simulink model "Traffic_Light_ROS2_demo"  (R2024b)
settings: Solver=FixedStepAuto  StartTime=0.0  StopTime=60  FixedStep=0.1  MaxStep=0.05  RelTol=1e-3
model workspace (MAT data in the model file):
  SL_ROS_VariableLengthArrays_MaxSizes : object (value not decoded)
undefined symbols (not defined in the file or in its folder): brake, gear, hand_brake, manual_gear_shift, reverse, steer, throttle
libraries: ros2lib x9, visionsinks x1
(part 2 of 2)

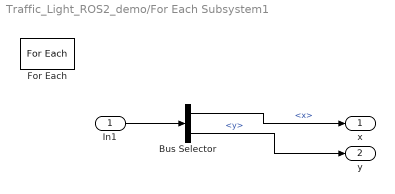
== system Traffic_Light_ROS2_demo/For Each Subsystem1 ==
  In1 : Inport  Partition=on  PartitionDimension=1  PartitionWidth=1  PartitionOffset=0
  Bus Selector : BusSelector  OutputSignals=pose.position.x,pose.position.y
  For Each : ForEach  DisableCoverage=on
  x : Outport  ConcatenationDimension=1
  y : Outport  Port=2  ConcatenationDimension=1
  wires:
  In1/1 -> Bus Selector/1
  Bus Selector/1 -> x/1  "<x>"
  Bus Selector/2 -> y/1  "<y>"

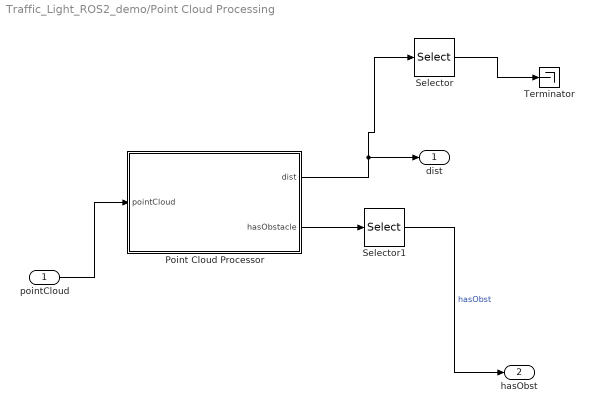
== system Traffic_Light_ROS2_demo/Point Cloud Processing ==
  pointCloud : Inport
  Point Cloud Processor : MATLAB Function  TreatAsAtomicUnit=on
  Selector : Selector  InputPortWidth=10000  IndexOptions=Index vector (dialog)  Indices=1  OutputSizes=1
  Selector1 : Selector  IndexOptions=Index vector (dialog)  Indices=1  OutputSizes=1
  Terminator : Terminator
  dist : Outport
  hasObst : Outport  Port=2
  wires:
  Point Cloud Processor/2(hasObstacle) -> Selector1/1
  Selector/1 -> Terminator/1
  pointCloud/1 -> Point Cloud Processor/1(pointCloud)
  Point Cloud Processor/1(dist) -> dist/1, Selector/1
  Selector1/1 -> hasObst/1  "hasObst"

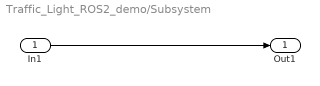
== system Traffic_Light_ROS2_demo/Subsystem ==
  In1 : Inport
  Out1 : Outport
  wires:
  In1/1 -> Out1/1

== matlab function Traffic_Light_ROS2_demo/Point Cloud Processing/Point Cloud Processor ==
  data: pointCloud input; dist output size=[10000,1]; hasObstacle output double
function [dist, hasObstacle] = detectObstacles(pointCloud)
% Detect obstacles from a point cloud and calculate the closest distance.

% Inputs:
%   pointCloud - Nx3 array of [x, y, z] points (point cloud data)
%   lateralRange - Lateral range of interest (meters)
%   zGroundThreshold - Minimum z-value to exclude ground points (meters)

% Outputs:
%   dist - Closest distance to an obstacle (scalar, meters)
%   hasObstacle - Boolean flag indicating if an obstacle is detected

% Initialize outputs
dist = single(inf); % Default to infinity
hasObstacle = 0;


% Check if pointCloud is empty
if isempty(pointCloud)
    return; % Return default outputs
end

% Extract coordinates
x = pointCloud(:, 1); % Forward (X) axis
y = pointCloud(:, 2); % Lateral (Y) axis
z = pointCloud(:, 3); % Vertical (Z) axis

lateralRange = 3;
zGroundThreshold = -2;

% Filter points within region of interest (ROI)
% ROI Criteria:
% - In front of the ego vehicle: x > 0
% - Within lateral range: |y| < lateralRange
% - Above ground: z > zGroundThreshold
isInROI = (x > 0) & (abs(y) < lateralRange) & (z > zGroundThreshold);

% Apply filter
filteredPoints = pointCloud(isInROI, :);

% Compute the closest distance
if ~isempty(filteredPoints)
    % Compute Euclidean distances in the X-Y plane
    % distances = sqrt(filteredPoints(:, 1).^2 + filteredPoints(:, 2).^2); 
    % dist = min(distances); % Find the closest distance
    dist = mean(filteredPoints(:, 1));
    hasObstacle = 1; % Set obstacle flag to true
end

end

== matlab function Traffic_Light_ROS2_demo/Visualize Point cloud2 ==
  data: xyzPoints input
function VisualizePointCloud(xyzPoints)
%VisualizePointCloud Display point cloud

coder.extrinsic('isOpen', 'pcplayer')

persistent player;

if isempty(player)
    % Configure axes limits
    xlimits = [-90 90];
    ylimits = [-90 90];
    zlimits = [ -5 40];
    
    % Create a streaming Lidar viewer
    player = pcplayer(xlimits, ylimits, zlimits);
end

if ~isempty(player) && isOpen(player)
    view(player, xyzPoints);
end

== matlab function Traffic_Light_ROS2_demo/MATLAB Function3 ==
  data: waypointsX input; waypointsX_local output; waypointsY input; vehicleX input; vehicleY input; vehicleYaw input; waypointsY_local output; Curvature output; CurvatureDerivative output; HeadingAngle output; LateralOffset output
function [waypointsX_local, waypointsY_local, Curvature, CurvatureDerivative, HeadingAngle, LateralOffset] = computeLaneCenter(waypointsX, waypointsY, vehicleX, vehicleY, vehicleYaw)
    % Inputs:
    %   waypointsX: X coordinates of the waypoints (Nx1 vector)
    %   waypointsY: Y coordinates of the waypoints (Nx1 vector)
    %   vehicleX: X coordinate of the vehicle
    %   vehicleY: Y coordinate of the vehicle
    %   vehicleYaw: Vehicle orientation (yaw) in radians
    % Outputs:
    %   Curvature: Lane curvature at the vehicle's position
    %   CurvatureDerivative: Rate of change of curvature
    %   HeadingAngle: Lane heading angle at the vehicle's position
    %   LateralOffset: Distance from the vehicle to the lane center (meters)

    % Ensure inputs are column vectors
    waypointsX = waypointsX(:);
    waypointsY = waypointsY(:);

    % Transform waypoints to local vehicle coordinates
    dx = waypointsX - vehicleX;
    dy = waypointsY - vehicleY;
    waypointsX_local = dx * cos(vehicleYaw) + dy * sin(vehicleYaw);
    waypointsY_local = -dx * sin(vehicleYaw) + dy * cos(vehicleYaw);

    % Filter waypoints to include only those ahead of the vehicle
    maxRange = 25; % Limit to 50 meters ahead
    rangeIdx = waypointsX_local > 0 & waypointsX_local < maxRange;
    waypointsX_local = waypointsX_local(rangeIdx);
    waypointsY_local = waypointsY_local(rangeIdx);

    % Ensure enough points are available for fitting
    if numel(waypointsX_local) < 3
        % Not enough points to compute reliably
        Curvature = single(0);
        CurvatureDerivative = single(0);
        HeadingAngle = single(0);
        LateralOffset = single(0);
        return;
    end

    % Fit a 2nd-order polynomial to the filtered waypoints
    polyCoeffs = polyfit(waypointsX_local, waypointsY_local, 2); % y = ax^2 + bx + c
    a = polyCoeffs(1); % Quadratic coefficient
    b = polyCoeffs(2); % Linear coefficient
    c = polyCoeffs(3); % Constant term

    % Curvature: k = 2a / (1 + b^2)^(3/2)
    Curvature = single(2 * a / (1 + b^2)^(3/2));

    % Curvature Derivative: k' = -6a^2b / (1 + b^2)^(5/2)
    CurvatureDerivative = single(-6 * a^2 * b / (1 + b^2)^(5/2));

    % Heading Angle: theta = atan(b)
    HeadingAngle = single(atan(b));

    % Lateral Offset: y = ax^2 + bx + c at x = 0
    LateralOffset = single(c); % Since x_vehicle_local = 0
    % 
    % % Debugging Outputs (optional)
    % disp('Polynomial Coefficients (a, b, c):');
    % disp(polyCoeffs);
    % disp('Curvature:');
    % disp(Curvature);
    % disp('Curvature Derivative:');
    % disp(CurvatureDerivative);
    % disp('Heading Angle:');
    % disp(HeadingAngle);
    % disp('Lateral Offset:');
    % disp(LateralOffset);
end

== matlab function Traffic_Light_ROS2_demo/MATLAB Function6 ==
  data: qx input; yaw output; qy input; qz input; qw input
function yaw = quaternionToYaw(qx, qy, qz, qw)
    % Convert quaternion (qx, qy, qz, qw) to yaw angle in radians
    % This formula is based on the standard conversion from quaternion to Euler angles

    % Calculate yaw from quaternion
    siny_cosp = 2 * (qw * qz + qx * qy);
    cosy_cosp = 1 - 2 * (qy^2 + qz^2);
    yaw = atan2(siny_cosp, cosy_cosp); % result is in radians
end
